simulink model "BasicHeadDemo"  (Simulink 6.2)
settings: Solver=ode45  StartTime=0.0  StopTime=10.0  RelTol=1e-3
settings Model: LastModifiedBy=suarezjl
settings DataIOCC: SignalLoggingName=sigsOut
settings HardwareCC: TargetUnknown=on

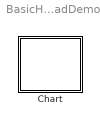
== system BasicHeadDemo ==
  Chart : Stateflow chart

== stateflow chart Chart ==
  state StartCameras
    \\Sally\LeftCameraAgent\StateMachine.LoadSM()
    \\Sally\LeftCameraAgent\StateMachine.Start()
    \\Sally\RightCameraAgent\StateMachine.LoadSM()
    \\Sally\RightCameraAgent\StateMachine.Start()
  state StartHead
    \\Sally\HeadAgent\StateMachine.LoadSM()
    \\Sally\HeadAgent\StateMachine.Start()
  state Stop
    \\Sally\HeadAgent\StateMachine.Stop()
    \\Sally\LeftCameraAgent\StateMachine.Stop()
    \\Sally\RightCameraAgent\StateMachine.Stop()
  (default) -> StartCameras : Start
  StartCameras -> StartHead : Always
  StartHead -> Stop : Signal="Stop"
